simulink model "sieving"  (R2022b)
settings: Solver=VariableStepAuto  StartTime=0.0  StopTime=10  RelTol=1e-3
settings Model: Creator=Sulith  LastModifiedBy=Sulith

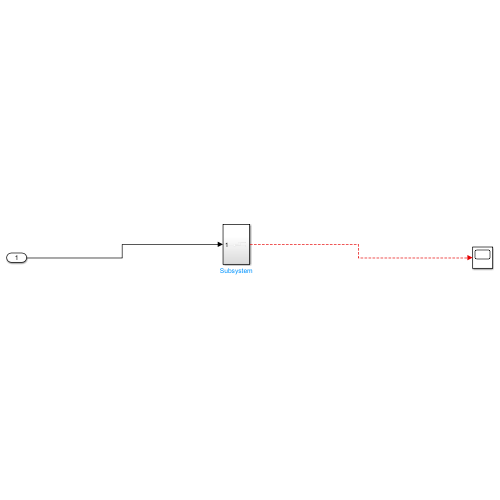
[thumbnail: Simulink's stored preview of the top-level diagram]
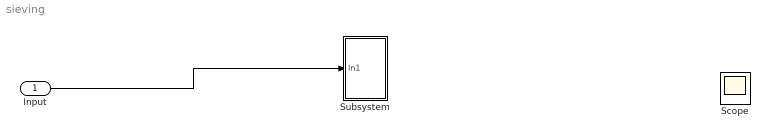
== system sieving ==
  Input : Inport
  Scope : Scope
  Subsystem : Subsystem
  wires:
  Input/1 -> Subsystem/1(In1)
  ? -> Scope/1

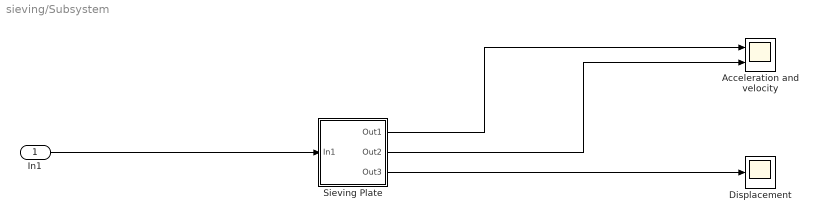
== system sieving/Subsystem ==
  In1 : Inport
  Acceleration and velocity : Scope  NumInputPorts=2
  Displacement : Scope
  Sieving Plate : Subsystem
  wires:
  In1/1 -> Sieving Plate/1(In1)
  Sieving Plate/1(Out1) -> Acceleration and velocity/1
  Sieving Plate/2(Out2) -> Acceleration and velocity/2
  Sieving Plate/3(Out3) -> Displacement/1

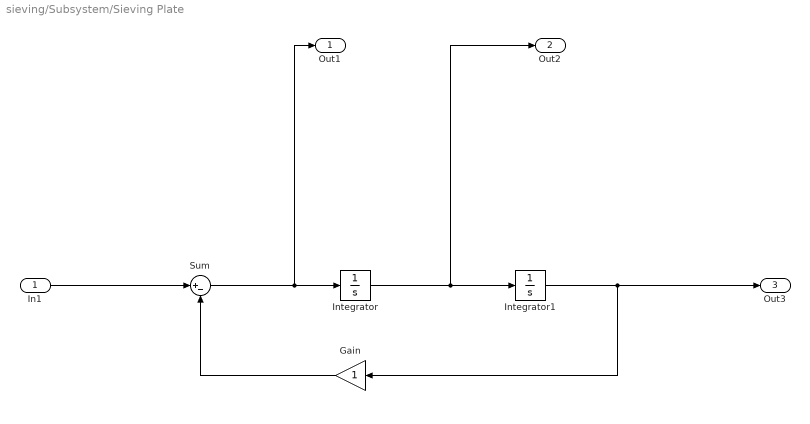
== system sieving/Subsystem/Sieving Plate ==
  In1 : Inport
  Gain : Gain
  Integrator : Integrator  InitialCondition=5
  Integrator1 : Integrator
  Sum : Sum  Inputs=|+-
  Out1 : Outport
  Out2 : Outport  Port=2
  Out3 : Outport  Port=3
  wires:
  In1/1 -> Sum/1
  Integrator1/1 -> Out3/1, Gain/1
  Sum/1 -> Out1/1, Integrator/1
  Gain/1 -> Sum/2
  Integrator/1 -> Out2/1, Integrator1/1
